simulink model "Validacion_modelo"  (R2021b)
settings: Solver=VariableStepAuto  StartTime=0.0  StopTime=10.0  RelTol=1e-3
settings Model: Creator=juanse  LastModifiedBy=juanse

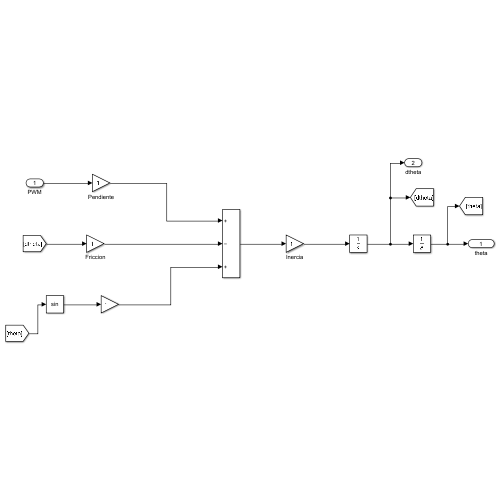
[thumbnail: Simulink's stored preview of the top-level diagram]
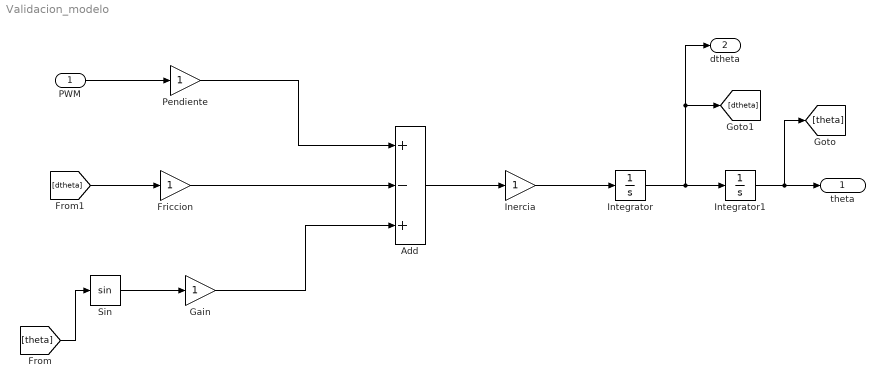
== system Validacion_modelo ==
  PWM : Inport
  Add : Sum  Inputs=+-+
  Friccion : Gain
  Gain : Gain
  Inercia : Gain
  Integrator : Integrator
  Integrator1 : Integrator
  Pendiente : Gain
  Sin : Trigonometry
  theta : Outport
  dtheta : Outport  Port=2
  wires:
  [theta] -> Sin/1
  Sin/1 -> Gain/1
  Gain/1 -> Add/3
  [dtheta] -> Friccion/1
  Friccion/1 -> Add/2
  PWM/1 -> Pendiente/1
  Pendiente/1 -> Add/1
  Add/1 -> Inercia/1
  Inercia/1 -> Integrator/1
  Integrator/1 -> [dtheta], dtheta/1, Integrator1/1
  Integrator1/1 -> [theta], theta/1
